simulink model "findClosestTrajectoryIndex"  (R2024a)
settings: Solver=VariableStepAuto  StartTime=0.0  StopTime=10.0  RelTol=1e-3
undefined symbols (not defined in the file): T
settings Model: Creator=matlab.cut  LastModifiedBy=matlab.cut

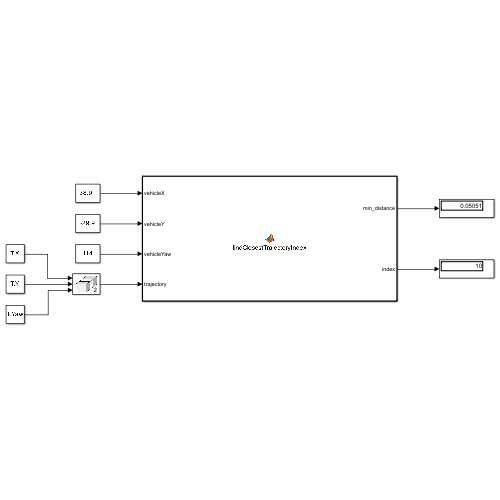
[thumbnail: Simulink's stored preview of the top-level diagram]
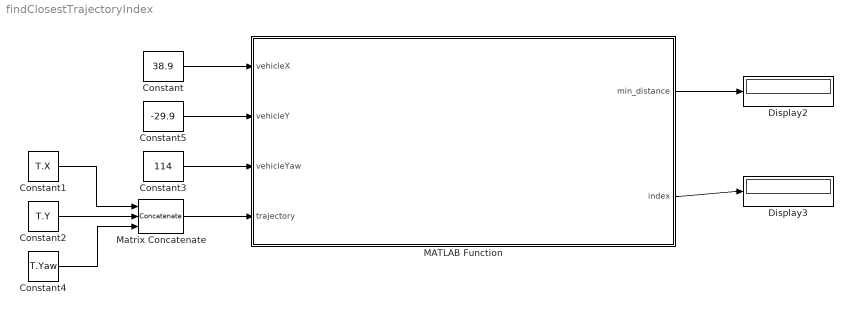
== system findClosestTrajectoryIndex ==
  Constant : Constant  Value=38.9
  Constant1 : Constant  Value=T.X
  Constant2 : Constant  Value=T.Y
  Constant3 : Constant  Value=114
  Constant4 : Constant  Value=T.Yaw
  Constant5 : Constant  Value=-29.9
  Display2 : Display
  Display3 : Display
  MATLAB Function : MATLAB Function  TreatAsAtomicUnit=on
  Matrix Concatenate : Concatenate  NumInputs=3  Mode=Multidimensional array  ConcatenateDimension=2
  wires:
  Constant1/1 -> Matrix Concatenate/1
  Constant2/1 -> Matrix Concatenate/2
  Matrix Concatenate/1 -> MATLAB Function/4(trajectory)
  Constant4/1 -> Matrix Concatenate/3
  Constant3/1 -> MATLAB Function/3(vehicleYaw)
  Constant5/1 -> MATLAB Function/2(vehicleY)
  Constant/1 -> MATLAB Function/1(vehicleX)
  MATLAB Function/1(min_distance) -> Display2/1
  MATLAB Function/2(index) -> Display3/1

== matlab function findClosestTrajectoryIndex/MATLAB Function ==
  data: vehicleX input; vehicleY input; vehicleYaw input; trajectory input; min_distance output; index output
function [min_distance, index] = findClosestTrajectoryIndex(vehicleX, vehicleY, vehicleYaw, trajectory)
    % trajectory é uma matriz Nx3 onde cada linha representa [X, Y, Yaw]

    % Inicializa as variáveis para armazenar a menor distância e o ponto mais próximo
    min_distance = inf;
    index = 0;
    %closest_point = [];
    
    % Converte a diferença de YAW para radianos
    yaw_diff_threshold = deg2rad(20);
    
    % Itera sobre cada ponto na trajetória
    for i = 1:size(trajectory, 1)
        % Coordenadas e YAW do ponto atual da trajetória
        pointX = trajectory(i, 1);
        pointY = trajectory(i, 2);
        pointYaw = trajectory(i, 3);
        
        % Calcula a distância euclidiana entre o veículo e o ponto atual
        distance = sqrt((vehicleX - pointX)^2 + (vehicleY - pointY)^2);
        
        % Calcula a diferença de YAW entre o veículo e o ponto atual
        yaw_diff = abs(deg2rad(vehicleYaw) - deg2rad(pointYaw));
        
        % Ajusta yaw_diff para estar no intervalo [0, pi]
        yaw_diff = mod(yaw_diff, 2*pi);
        if yaw_diff > pi
            yaw_diff = 2*pi - yaw_diff;
        end
        
        % Verifica se a diferença de YAW está dentro do limite de 20 graus
        if yaw_diff < yaw_diff_threshold
            % Atualiza a menor distância e o ponto mais próximo se este ponto for mais próximo
            if distance < min_distance
                min_distance = distance;
                %closest_point = [pointX, pointY, pointYaw];
                index = i;
            end
        end
    end
end
